simulink model "WeatherCondition_integrated"  (R2020a)
settings: Solver=VariableStepAuto  StartTime=0.0  StopTime=10.0  RelTol=1e-3
values from neighbouring files (symbols this model uses):
  Ignition : value not decoded    [ALS_Project_dd.sldd]
  Weather : value not decoded    [ALS_Project_dd.sldd]
undefined symbols (not defined in the file or in its folder): AlsMode
libraries: simulink x12
settings Model: Creator=Pratik shinde  LastModifiedBy=Pratik shinde
settings ConfigComp: DVTestSuiteOptimization=Auto  DVDetectOutOfBounds=on

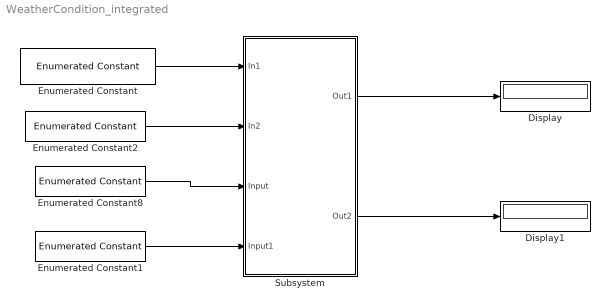
== system WeatherCondition_integrated ==
  Display : Display
  Display1 : Display
  Enumerated Constant : simulink/Sources/Enumerated Constant  OutDataTypeStr=Enum: Weather  Value=Weather.Rain_detected  SampleTime=inf
  Enumerated Constant1 : simulink/Sources/Enumerated Constant  OutDataTypeStr=Enum: AlsMode  Value=AlsMode.On  SampleTime=inf
  Enumerated Constant2 : simulink/Sources/Enumerated Constant  OutDataTypeStr=Enum: Weather  Value=Weather.Fog_detected  SampleTime=inf
  Enumerated Constant8 : simulink/Sources/Enumerated Constant  OutDataTypeStr=Enum: Ignition  Value=Ignition.On  SampleTime=inf
  Subsystem : Subsystem
  wires:
  Enumerated Constant/1 -> Subsystem/1(In1)
  Enumerated Constant2/1 -> Subsystem/2(In2)
  Subsystem/1(Out1) -> Display/1
  Subsystem/2(Out2) -> Display1/1
  Enumerated Constant8/1 -> Subsystem/3(Input)
  Enumerated Constant1/1 -> Subsystem/4(Input1)

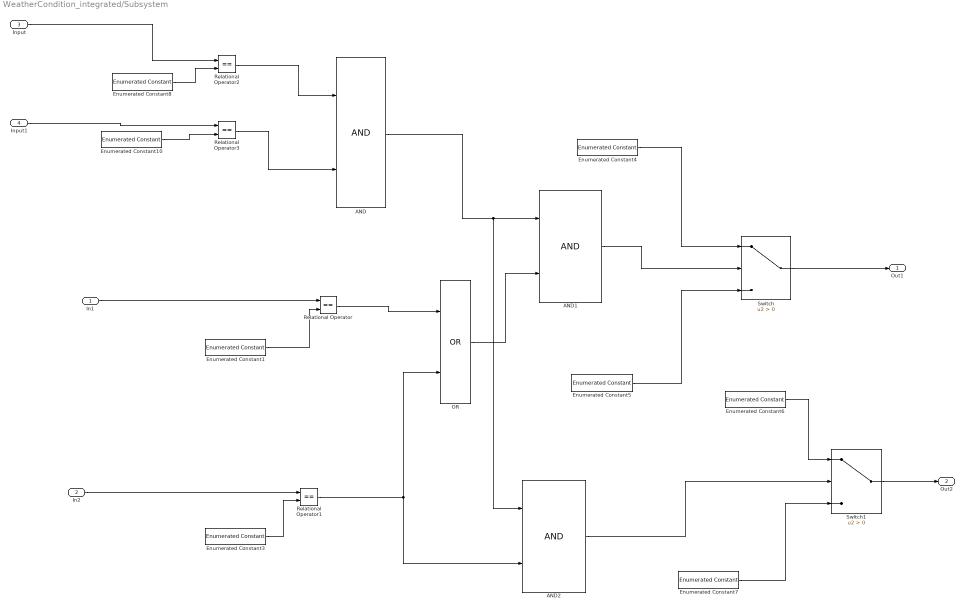
== system WeatherCondition_integrated/Subsystem ==
  In1 : Inport
  In2 : Inport  Port=2
  Input : Inport  Port=3
  Input1 : Inport  Port=4
  AND : Logic  AllPortsSameDT=off  OutDataTypeStr=boolean
  AND1 : Logic  AllPortsSameDT=off  OutDataTypeStr=boolean
  AND2 : Logic  AllPortsSameDT=off  OutDataTypeStr=boolean
  Enumerated Constant1 : simulink/Sources/Enumerated Constant  OutDataTypeStr=Enum: Weather  Value=Weather.Rain_detected  SampleTime=inf
  Enumerated Constant10 : simulink/Sources/Enumerated Constant  OutDataTypeStr=Enum: AlsMode  Value=AlsMode.On  SampleTime=inf
  Enumerated Constant3 : simulink/Sources/Enumerated Constant  OutDataTypeStr=Enum: Weather  Value=Weather.Fog_detected  SampleTime=inf
  Enumerated Constant4 : simulink/Sources/Enumerated Constant  OutDataTypeStr=Enum: Weather  Value=Weather.Lowbeam_On  SampleTime=inf
  Enumerated Constant5 : simulink/Sources/Enumerated Constant  OutDataTypeStr=Enum: Weather  Value=Weather.Head_light_off  SampleTime=inf
  Enumerated Constant6 : simulink/Sources/Enumerated Constant  OutDataTypeStr=Enum: Weather  Value=Weather.FogLight_On  SampleTime=inf
  Enumerated Constant7 : simulink/Sources/Enumerated Constant  OutDataTypeStr=Enum: Weather  Value=Weather.FogLight_Off  SampleTime=inf
  Enumerated Constant8 : simulink/Sources/Enumerated Constant  OutDataTypeStr=Enum: Ignition  Value=Ignition.On  SampleTime=inf
  OR : Logic  Operator=OR  AllPortsSameDT=off  OutDataTypeStr=boolean
  Relational Operator{,1..3} (4 alike) : RelationalOperator  Operator===  OutDataTypeStr=boolean  RndMeth=Simplest
  Switch : Switch  Criteria=u2 > Threshold
  Switch1 : Switch  Criteria=u2 > Threshold
  Out1 : Outport
  Out2 : Outport  Port=2
  wires:
  Enumerated Constant1/1 -> Relational Operator/2
  Enumerated Constant7/1 -> Switch1/3
  Enumerated Constant3/1 -> Relational Operator1/2
  In2/1 -> Relational Operator1/1
  Enumerated Constant5/1 -> Switch/3
  Enumerated Constant6/1 -> Switch1/1
  Enumerated Constant4/1 -> Switch/1
  Relational Operator1/1 -> AND2/2, OR/2
  Switch1/1 -> Out2/1
  In1/1 -> Relational Operator/1
  Switch/1 -> Out1/1
  Relational Operator/1 -> OR/1
  Input/1 -> Relational Operator2/1
  Enumerated Constant8/1 -> Relational Operator2/2
  Enumerated Constant10/1 -> Relational Operator3/2
  Relational Operator2/1 -> AND/1
  Relational Operator3/1 -> AND/2
  AND/1 -> AND2/1, AND1/1
  OR/1 -> AND1/2
  AND1/1 -> Switch/2
  Input1/1 -> Relational Operator3/1
  AND2/1 -> Switch1/2
